simulink model "OSC"  (R2017b)
settings: Solver=FixedStepAuto  StartTime=0.0  StopTime=stopTime  FixedStep=stepSize  RelTol=1e-3
values from neighbouring files (symbols this model uses):
  mu = 398600    [AA279D_FINAL.m]    (also in AA279D_PSET1.m; AA279D_PSET2.m; AA279D_PSET2_a_change.m; AA279D_PSET3.m)
  r_eci2 = r_eci2'    [AA279D_PSET1.m]
  v_eci2 = v_eci2'    [AA279D_PSET1.m]
settings Model: Creator=cwcovert  LastModifiedBy=cwcovert

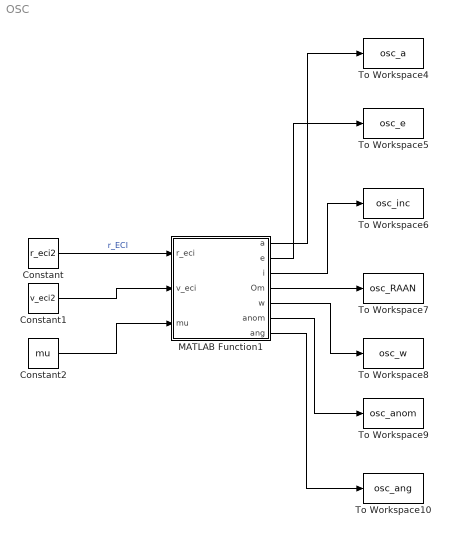
== system OSC ==
  Constant : Constant  Value=r_eci2
  Constant1 : Constant  Value=v_eci2
  Constant2 : Constant  Value=mu
  MATLAB Function1 : MATLAB Function  TreatAsAtomicUnit=on
  To Workspace10 : ToWorkspace  VariableName=osc_ang  SampleTime=-1
  To Workspace4 : ToWorkspace  VariableName=osc_a  SampleTime=-1
  To Workspace5 : ToWorkspace  VariableName=osc_e  SampleTime=-1
  To Workspace6 : ToWorkspace  VariableName=osc_inc  SampleTime=-1
  To Workspace7 : ToWorkspace  VariableName=osc_RAAN  SampleTime=-1
  To Workspace8 : ToWorkspace  VariableName=osc_w  SampleTime=-1
  To Workspace9 : ToWorkspace  VariableName=osc_anom  SampleTime=-1
  wires:
  MATLAB Function1/3(i) -> To Workspace6/1
  MATLAB Function1/6(anom) -> To Workspace9/1
  Constant/1 -> MATLAB Function1/1(r_eci)  "r_ECI"
  MATLAB Function1/5(w) -> To Workspace8/1
  MATLAB Function1/7(ang) -> To Workspace10/1
  MATLAB Function1/2(e) -> To Workspace5/1
  MATLAB Function1/4(Om) -> To Workspace7/1
  MATLAB Function1/1(a) -> To Workspace4/1
  Constant1/1 -> MATLAB Function1/2(v_eci)
  Constant2/1 -> MATLAB Function1/3(mu)

== matlab function OSC/MATLAB Function1 ==
  data: r_eci input; a output; v_eci input; e output; mu input; i output; Om output; w output; anom output; ang output
function [a, e, i, Om, w, anom, ang] = ECI2OE(r_eci, v_eci, mu)
% ECI2OE Converts r and v in the ECI frame to orbital elements
%
% Inputs:
%   r_eci - 3x1 vector of radius in ECI frame [km]
%   v_eci - 3x1 vector of velocity in ECI frame [km]
%   mu    - gravitational parameter of central body [km^3/s^2]
%
% Outputs:
%   p     - semi-lactus rectum of orbit [km]
%   a     - semi-major axis of orbit [km]
%   e     - eccentricity of orbit
%   i     - inclination of orbit [deg]
%   Om    - right ascension of the ascending node [deg]
%   w     - argument of periapsis [deg]
%   v     - true anomaly [deg]
%   ang   - extra placeholder angle for special cases [deg]
%
% This function is able to handle any orbit type, including equatorial and
% circular orbits. The output ang will output the following values for each
% orbit type
%   1) Elliptical equatorial
%       Longitude of periapsis, Pi = Om + w
%   2) Circular inclined
%       Argument of latitude, u = w + anom
%   3) Circular equatorial
%       True latitude, lambda = Om + w + anom
% Otherwise, ang will be undefined (NaN)

r = norm(r_eci);
v = norm(v_eci);

% Create all necessary vectors
hVec = cross(r_eci, v_eci);
h = norm(hVec);

nVec = cross([0, 0, 1], hVec);
n = norm(nVec);

eVec = (1/mu)*((v^2 - mu/r)*r_eci - dot(r_eci, v_eci)*v_eci);
e = norm(eVec);

% Compute the size of the orbit
mechEnergy = 0.5*v^2 - mu/r;

if e ~= 1
    a = -mu/(2*mechEnergy);
else
    a = inf; % Semi-major axis undefined for parabolas
end

% Compute the orientation of the orbit
i = rad2deg(acos(hVec(3)/h));
Om = rad2deg(acos(nVec(1)/n));
w = rad2deg(acos(dot(nVec, eVec)/(n*e)));
anom = rad2deg(acos(dot(eVec, r_eci)/(e*r)));

% Place angles in the correct domains
if nVec(2) < 0
    Om = 360 - Om;
end
if eVec(3) < 0
    w = 360 - w;
end
if dot(r_eci, v_eci) < 0
    anom = 360 - anom;
end

% Account for any special cases
if i == 0 && e ~= 0 % Elliptical equatorial
    % Provide the longitude of periapsis (PI = Om + w)
    ang = rad2deg(acos(eVec(1)/e));

    if eVec(2) < 0
        ang = 360 - ang;
    end
elseif i ~= 0 && e == 0 % Circular inclined
    % Provide the argument of latitude (u = w + anom)
    ang = rad2deg(acos(dot(nVec, r_eci)/(n*r)));

    if r_eci(3) < 0
        ang = 360 - ang;
    end
elseif i == 0 && e == 0 % Circular equatorial
    % Provide the true latitude (lambda = Om + w + anom)
    ang = rad2deg(acos(r_eci(1)/r));

    if r_eci(2) < 0
        ang = 360 - ang;
    end
else
    % Default output for ang
    ang = NaN;
end
end
